simulink model "sgMdl_DNP3_1Client_1Server"  (R2024b)
settings: Solver=FixedStepAuto  StartTime=0.0  StopTime=inf  RelTol=1e-3  EnableMultiTasking=on
libraries: simulink x15, speedgoatlib_dnp3 x13
Description:
  | DNP3 - Loopback
settings Model: sg_rtwmakecfg_data=_sg_IO75X_v1_2_0__sg_netxLib_MSVC140_  ModifiedByFormat=Speedgoat  SimulationMode=external  Creator=Speedgoat  LastModifiedBy=Speedgoat
settings SolverCC: ConcurrentTasks=on  AlgebraicLoopSolver=TrustRegion  PositivePriorityOrder=on  InsertRTBMode=Never (minimum delay)
settings DataIOCC: LimitDataPoints=on  SaveFormat=StructureWithTime  ReturnWorkspaceOutputs=off
settings OptimizationCC: BlockReduction=off  BooleanDataType=off  OptimizeBlockIOStorage=off  BufferReuse=off  GlobalBufferReuse=off  ExpressionFolding=off  LocalBlockOutputs=off  OptimizeDataStoreBuffers=off  BusAssignmentInplaceUpdate=off
settings DebuggingCC: SaveWithParameterizedLinksMsg=none  UnderspecifiedInitializationDetection=Classic  MergeDetectMultiDrivingBlocksExec=none  SignalResolutionControl=TryResolveAllWithWarning  TasksWithSamePriorityMsg=none  ParameterOverflowMsg=warning  UnconnectedInputMsg=warning  UnconnectedOutputMsg=warning  UnconnectedLineMsg=warning  SFUnexpectedBacktrackingDiag=warning  SFNoUnconditionalDefaultTransitionDiag=warning  SFExecutionAtInitializationDiag=none  ArithmeticOperatorsInVariantConditions=warning
settings HardwareCC: ProdBitPerLong=64  ProdLongLongMode=on  ProdHWDeviceType=Intel->x86-64 (Linux 64)  TargetBitPerPointer=64  TargetBitPerSizeT=64  TargetBitPerPtrDiffT=64  TargetLongLongMode=on  TargetIntDivRoundTo=Zero  TargetEndianess=LittleEndian  TargetWordSize=64  TargetHWDeviceType=MATLAB Host
settings ModelReferenceCC: EnableRefExpFcnMdlSchedulingChecks=on  PropagateSignalLabelsOutOfModel=off
settings SFSimCC: SimUseLocalCustomCode=off  CustomCodeUndefinedFunction=UseInterfaceOnly
settings RTWCC: Description=Speedgoat Real-Time Target Machine  SystemTargetFile=speedgoat.tlc  TemplateMakefile=slrealtime_default_tmf  RTWUseLocalCustomCode=off  Toolchain=Simulink Real-Time Toolchain  BuildConfiguration=Faster Runs  TargetLang=C++  GPUComputeCapability=3.5  DLArmComputeVersion=19.05
settings CodeAppCC: StateflowObjectComments=on
settings SimulinkRealTimeTargetCC: SubcomponentCodeInterfacePackaging=Reusable function  InstructionSetFMA=off  LogToMDFFile=off  SLRTFileLogMaxRuns=10
settings ConfigComp: CovMetricSettings=dw  CovSaveCumulativeToWorkspaceVar=on  CovSaveSingleToWorkspaceVar=on  CovExternalEMLEnable=off  CovBoundaryAbsTol=1.0e-5

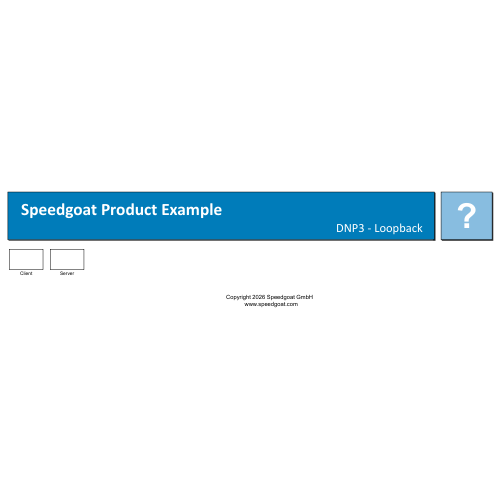
[thumbnail: Simulink's stored preview of the top-level diagram]
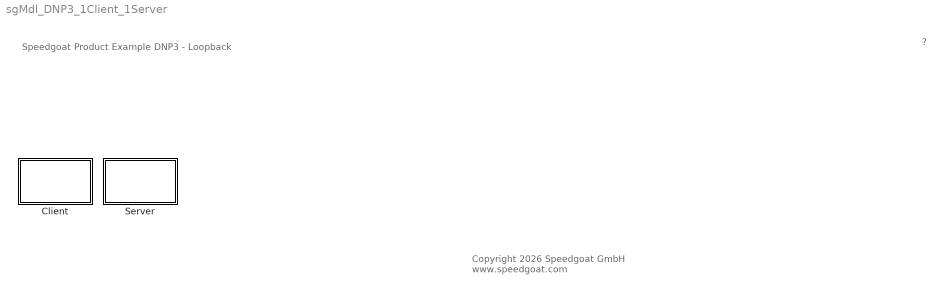
== system sgMdl_DNP3_1Client_1Server ==
  note: Speedgoat Product Example
      | DNP3 - Loopback
  note: ?
  note: Copyright 2026 Speedgoat GmbH
      |  www.speedgoat.com
  Client : Subsystem
  Server : Subsystem

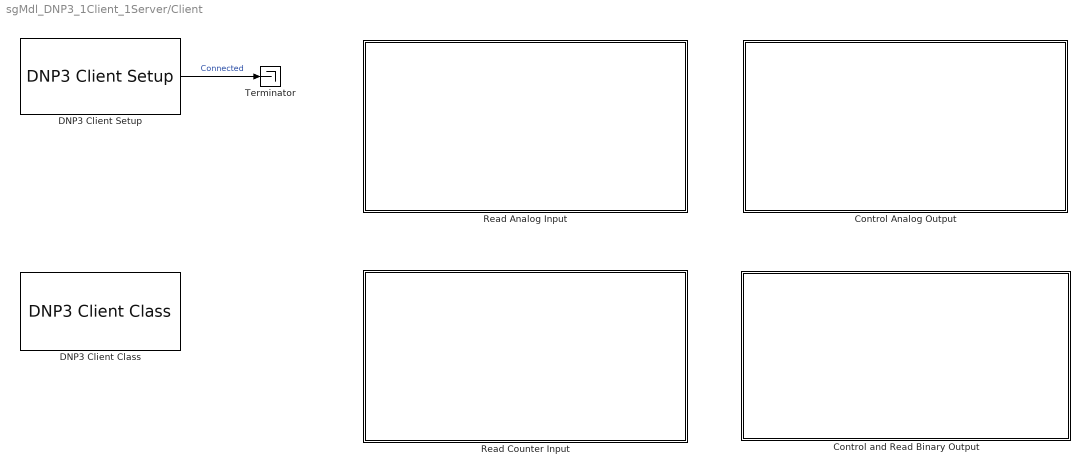
== system sgMdl_DNP3_1Client_1Server/Client ==
  Control Analog Output : Subsystem
  Control and Read Binary Output : Subsystem
  DNP3 Client Class : speedgoatlib_dnp3/Client/DNP3 Client Class  MasterID=0  OutstationID=1  SampleTime=-1  UnsolicitedClass0=off  UnsolicitedClass1=off  UnsolicitedClass2=off  UnsolicitedClass3=on  PollClass0=off  PollClass1=off  PollClass2=off  PollClass3=off  ClassTable={ '30 Analog input', '0', '1', 'Class 3' }
      settings: SourceProductName=DNP3
  DNP3 Client Setup : speedgoatlib_dnp3/Client/DNP3 Client Setup  NetworkID=0  MasterID=0  IpAddrStr='192.168.10.100'  KeepAlive=10000  RxTimeout=50  DataLinkRetries=3  SampleTime=0.001  OutstationTable={ '1', '192.168.10.101', '20000' }
      settings: SourceProductName=DNP3
  Read Analog Input : Subsystem
  Read Counter Input : Subsystem
  Terminator : Terminator
  wires:
  DNP3 Client Setup/1 -> Terminator/1  "Connected"

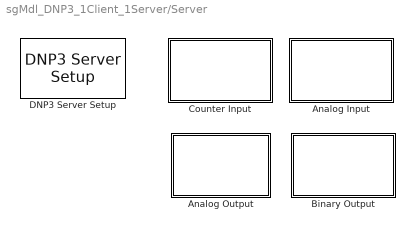
== system sgMdl_DNP3_1Client_1Server/Server ==
  Analog Input : Subsystem
  Analog Output : Subsystem
  Binary Output : Subsystem
  Counter Input : Subsystem
  DNP3 Server Setup : speedgoatlib_dnp3/Server/DNP3 Server Setup  OutstationID=1  IpAddrStr='192.168.10.101'  TcpPort=20000  Deadband=1.5  DevAttrCell={}  NumBinInPoints=8  NumBinInEvents=100  NumDBinInPoints=8  NumDBinInEvents=100  NumCntInPoints=8  NumCntInEvents=100  NumAnalogInPoints=8  NumAnalogInEvents=100  NumBinOutPoints=8  NumBinOutEvents=100  NumAnalogOutPoints=8  NumAnalogOutEvents=100
      settings: SourceProductName=DNP3

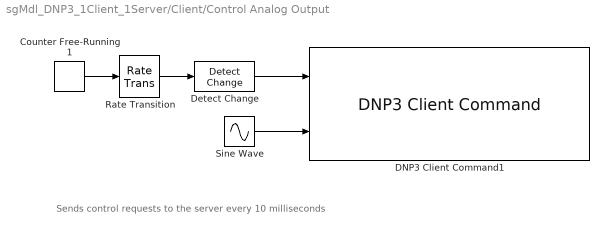
== system sgMdl_DNP3_1Client_1Server/Client/Control Analog Output ==
  note: Sends control requests to the server every 10 milliseconds
  Counter Free-Running1 : simulink/Sources/Counter Free-Running  NumBits=32  tsamp=0.01
  DNP3 Client Command1 : speedgoatlib_dnp3/Client/DNP3 Client Command  MasterID=0  OutstationID=1  CommandMode=Dropdown  CommandDropDown=41:04:05 Control analog output (64-bit float)  CommandEdit=[41 4 5]  Index=0  Quantity=1  SampleTime=0.001
      settings: AttributesFormatString=%<CommandDropdown>  SourceProductName=DNP3
  Detect Change : simulink/Logic and Bit Operations/Detect Change  vinit=0  OutDataTypeStr=boolean
  Rate Transition : RateTransition
  Sine Wave : Sin  SineType=Sample based  Amplitude=10  Samples=2000  SampleTime=0.001
  wires:
  Detect Change/1 -> DNP3 Client Command1/1
  Sine Wave/1 -> DNP3 Client Command1/2
  Counter Free-Running1/1 -> Rate Transition/1
  Rate Transition/1 -> Detect Change/1

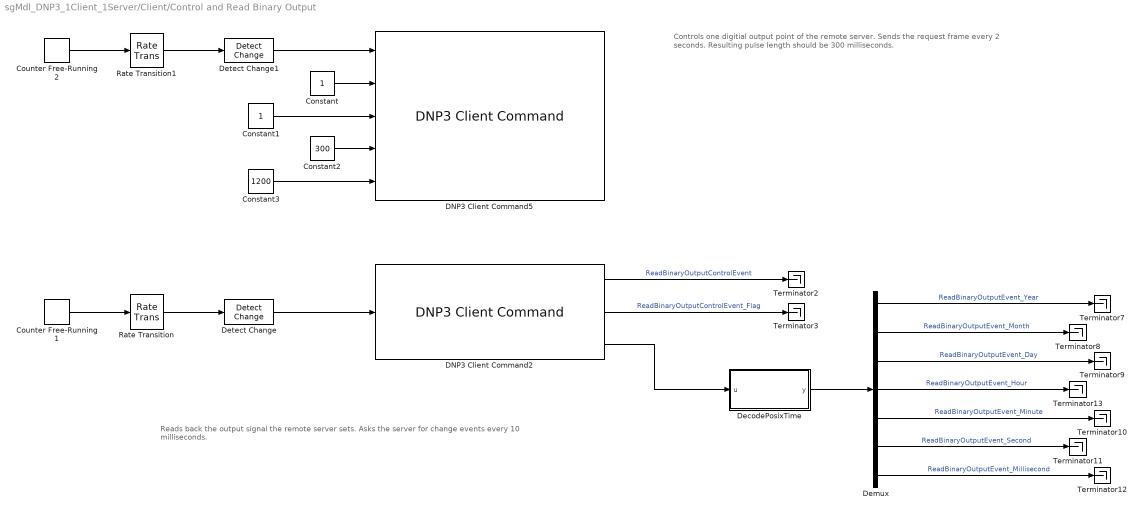
== system sgMdl_DNP3_1Client_1Server/Client/Control and Read Binary Output ==
  note: Controls one digitial output point of the remote server. Sends the request frame every 2 seconds. Resulting pulse length should be 300 milliseconds.
  note: Reads back the output signal the remote server sets. Asks the server for change events every 10 milliseconds.
  Constant : Constant  OutDataTypeStr=Inherit: Inherit via back propagation
  Constant1 : Constant  OutDataTypeStr=Inherit: Inherit via back propagation
  Constant2 : Constant  Value=300  OutDataTypeStr=Inherit: Inherit via back propagation
  Constant3 : Constant  Value=1200  OutDataTypeStr=Inherit: Inherit via back propagation
  Counter Free-Running1 : simulink/Sources/Counter Free-Running  NumBits=32  tsamp=0.01
  Counter Free-Running2 : simulink/Sources/Counter Free-Running  NumBits=32  tsamp=2
  DNP3 Client Command2 : speedgoatlib_dnp3/Client/DNP3 Client Command  MasterID=0  OutstationID=1  CommandMode=Dropdown  CommandDropDown=11:02:01 Read binary output event with time  CommandEdit=[11 2 1]  Index=0  Quantity=1  SampleTime=0.001
      settings: AttributesFormatString=%<CommandDropdown>  SourceProductName=DNP3
  DNP3 Client Command5 : speedgoatlib_dnp3/Client/DNP3 Client Command  MasterID=0  OutstationID=1  CommandMode=Dropdown  CommandDropDown=12:01:05 Control Relay Output  CommandEdit=[12 1 5]  Index=0  Quantity=1  SampleTime=0.001
      settings: AttributesFormatString=%<CommandDropdown>  SourceProductName=DNP3
  DecodePosixTime : MATLAB Function  TreatAsAtomicUnit=on
  Demux : Demux  Outputs=7
  Detect Change : simulink/Logic and Bit Operations/Detect Change  vinit=0  OutDataTypeStr=boolean
  Detect Change1 : simulink/Logic and Bit Operations/Detect Change  vinit=0  OutDataTypeStr=boolean
  Rate Transition : RateTransition
  Rate Transition1 : RateTransition
  Terminator{2..3,7..13} (9 alike) : Terminator
  wires:
  Demux/4 -> Terminator13/1  "ReadBinaryOutputEvent_Hour"
  Detect Change1/1 -> DNP3 Client Command5/1
  Constant1/1 -> DNP3 Client Command5/3
  Rate Transition1/1 -> Detect Change1/1
  Demux/3 -> Terminator9/1  "ReadBinaryOutputEvent_Day"
  Demux/5 -> Terminator10/1  "ReadBinaryOutputEvent_Minute"
  Counter Free-Running2/1 -> Rate Transition1/1
  Rate Transition/1 -> Detect Change/1
  Constant3/1 -> DNP3 Client Command5/5
  Demux/1 -> Terminator7/1  "ReadBinaryOutputEvent_Year"
  Constant2/1 -> DNP3 Client Command5/4
  Constant/1 -> DNP3 Client Command5/2
  Demux/2 -> Terminator8/1  "ReadBinaryOutputEvent_Month"
  Counter Free-Running1/1 -> Rate Transition/1
  DecodePosixTime/1(y) -> Demux/1
  DNP3 Client Command2/1 -> Terminator2/1  "ReadBinaryOutputControlEvent"
  DNP3 Client Command2/2 -> Terminator3/1  "ReadBinaryOutputControlEvent_Flag"
  Demux/7 -> Terminator12/1  "ReadBinaryOutputEvent_Millisecond"
  DNP3 Client Command2/3 -> DecodePosixTime/1(u)
  Demux/6 -> Terminator11/1  "ReadBinaryOutputEvent_Second"
  Detect Change/1 -> DNP3 Client Command2/1

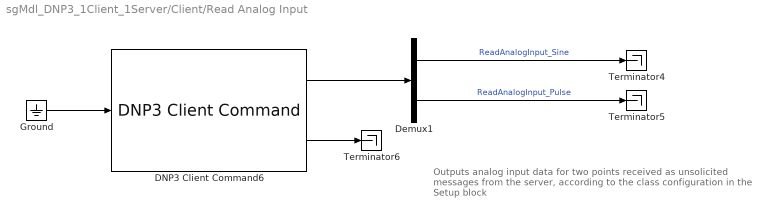
== system sgMdl_DNP3_1Client_1Server/Client/Read Analog Input ==
  note: Outputs analog input data for two points received as unsolicited messages from the server, according to the class configuration in the Setup block
  DNP3 Client Command6 : speedgoatlib_dnp3/Client/DNP3 Client Command  MasterID=0  OutstationID=1  CommandMode=Dropdown  CommandDropDown=32:06:01 Read analog input event with flag (64-bit float)  CommandEdit=[32 6 1]  Index=0  Quantity=2  SampleTime=0.001
      settings: AttributesFormatString=%<CommandDropdown>  SourceProductName=DNP3
  Demux1 : Demux  Outputs=2
  Ground : Ground
  Terminator4 : Terminator
  Terminator5 : Terminator
  Terminator6 : Terminator
  wires:
  Demux1/1 -> Terminator4/1  "ReadAnalogInput_Sine"
  Ground/1 -> DNP3 Client Command6/1
  Demux1/2 -> Terminator5/1  "ReadAnalogInput_Pulse"
  DNP3 Client Command6/2 -> Terminator6/1
  DNP3 Client Command6/1 -> Demux1/1

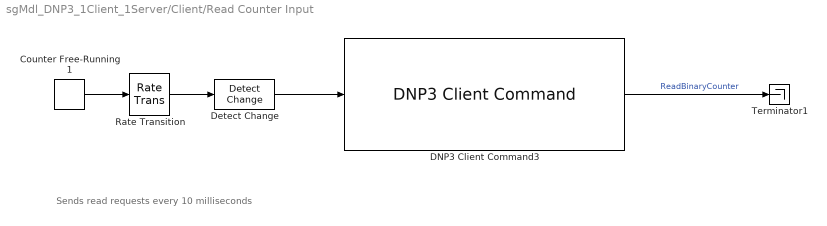
== system sgMdl_DNP3_1Client_1Server/Client/Read Counter Input ==
  note: Sends read requests every 10 milliseconds
  Counter Free-Running1 : simulink/Sources/Counter Free-Running  NumBits=32  tsamp=0.01
  DNP3 Client Command3 : speedgoatlib_dnp3/Client/DNP3 Client Command  MasterID=0  OutstationID=1  CommandMode=Dropdown  CommandDropDown=20:05:01 Read binary counter (32-bit integer)  CommandEdit=[20 5 1]  Index=0  Quantity=1  SampleTime=0.001
      settings: AttributesFormatString=%<CommandDropdown>  SourceProductName=DNP3
  Detect Change : simulink/Logic and Bit Operations/Detect Change  vinit=0  OutDataTypeStr=boolean
  Rate Transition : RateTransition
  Terminator1 : Terminator
  wires:
  DNP3 Client Command3/1 -> Terminator1/1  "ReadBinaryCounter"
  Detect Change/1 -> DNP3 Client Command3/1
  Counter Free-Running1/1 -> Rate Transition/1
  Rate Transition/1 -> Detect Change/1

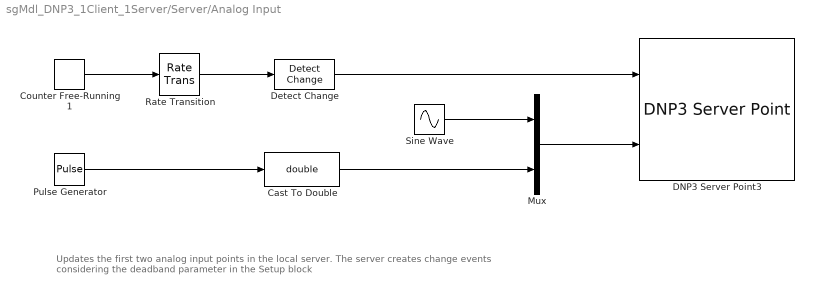
== system sgMdl_DNP3_1Client_1Server/Server/Analog Input ==
  note: Updates the first two analog input points in the local server. The server creates change events considering the deadband parameter in the Setup block
  Cast To Double : DataTypeConversion  OutDataTypeStr=double  SaturateOnIntegerOverflow=off  RndMeth=Floor
  Counter Free-Running1 : simulink/Sources/Counter Free-Running  NumBits=32  tsamp=0.01
  DNP3 Server Point3 : speedgoatlib_dnp3/Server/DNP3 Server Point  NetworkID=0  OutstationID=1  OperationMode=30 Write analog input  Length=2  SampleTime=0.001  Offset=0
      settings: AttributesFormatString=%<OperationMode>  SourceProductName=DNP3
  Detect Change : simulink/Logic and Bit Operations/Detect Change  vinit=0  OutDataTypeStr=boolean
  Mux : Mux  Inputs=2
  Pulse Generator : DiscretePulseGenerator  Amplitude=2  Period=1000  PulseWidth=500  SampleTime=0.001
  Rate Transition : RateTransition
  Sine Wave : Sin  SineType=Sample based  Amplitude=10  Samples=2000  SampleTime=0.001
  wires:
  Sine Wave/1 -> Mux/1
  Cast To Double/1 -> Mux/2
  Mux/1 -> DNP3 Server Point3/2
  Rate Transition/1 -> Detect Change/1
  Detect Change/1 -> DNP3 Server Point3/1
  Counter Free-Running1/1 -> Rate Transition/1
  Pulse Generator/1 -> Cast To Double/1

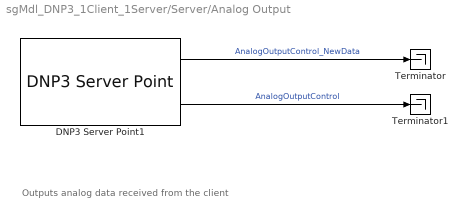
== system sgMdl_DNP3_1Client_1Server/Server/Analog Output ==
  note: Outputs analog data received from the client
  DNP3 Server Point1 : speedgoatlib_dnp3/Server/DNP3 Server Point  NetworkID=0  OutstationID=1  OperationMode=41 Indicate analog output control  Length=1  SampleTime=0.001  Offset=0
      settings: AttributesFormatString=%<OperationMode>  SourceProductName=DNP3
  Terminator : Terminator
  Terminator1 : Terminator
  wires:
  DNP3 Server Point1/2 -> Terminator1/1  "AnalogOutputControl"
  DNP3 Server Point1/1 -> Terminator/1  "AnalogOutputControl_NewData"

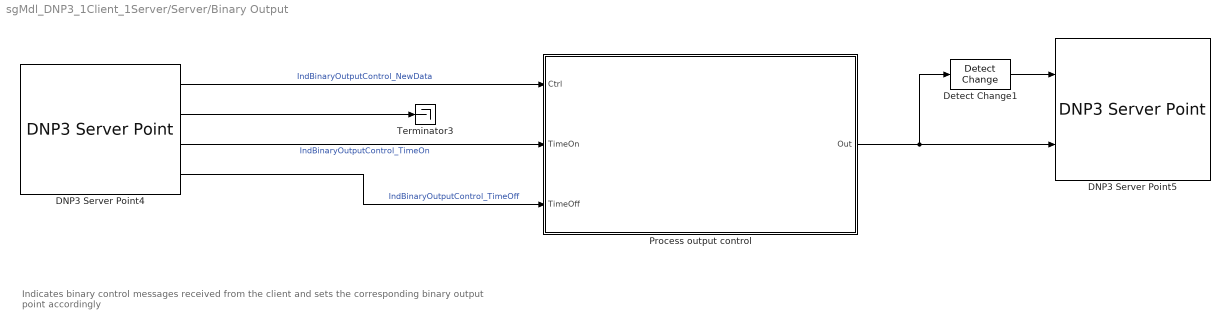
== system sgMdl_DNP3_1Client_1Server/Server/Binary Output ==
  note: Indicates binary control messages received from the client and sets the corresponding binary output point accordingly
  DNP3 Server Point4 : speedgoatlib_dnp3/Server/DNP3 Server Point  NetworkID=0  OutstationID=1  OperationMode=12 Indicate binary output control  Length=1  SampleTime=0.001  Offset=0
      settings: AttributesFormatString=%<OperationMode>  SourceProductName=DNP3
  DNP3 Server Point5 : speedgoatlib_dnp3/Server/DNP3 Server Point  NetworkID=0  OutstationID=1  OperationMode=10 Write binary output  Length=1  SampleTime=0.001  Offset=0
      settings: AttributesFormatString=%<OperationMode>  SourceProductName=DNP3
  Detect Change1 : simulink/Logic and Bit Operations/Detect Change  vinit=0  OutDataTypeStr=boolean
  Process output control : Subsystem
  Terminator3 : Terminator
  wires:
  DNP3 Server Point4/2 -> Terminator3/1
  DNP3 Server Point4/3 -> Process output control/2(TimeOn)  "IndBinaryOutputControl_TimeOn"
  DNP3 Server Point4/4 -> Process output control/3(TimeOff)  "IndBinaryOutputControl_TimeOff"
  Process output control/1(Out) -> Detect Change1/1, DNP3 Server Point5/2
  DNP3 Server Point4/1 -> Process output control/1(Ctrl)  "IndBinaryOutputControl_NewData"
  Detect Change1/1 -> DNP3 Server Point5/1

== system sgMdl_DNP3_1Client_1Server/Server/Counter Input ==
  note: Updates a local counter point
  Constant : Constant  OutDataTypeStr=Inherit: Inherit via back propagation
  Counter Free-Running : simulink/Sources/Counter Free-Running  NumBits=32  tsamp=0.001
  DNP3 Server Point2 : speedgoatlib_dnp3/Server/DNP3 Server Point  NetworkID=0  OutstationID=1  OperationMode=20 Write counter input  Length=1  SampleTime=0.001  Offset=0
      settings: AttributesFormatString=%<OperationMode>  SourceProductName=DNP3
  wires:
  Counter Free-Running/1 -> DNP3 Server Point2/2
  Constant/1 -> DNP3 Server Point2/1

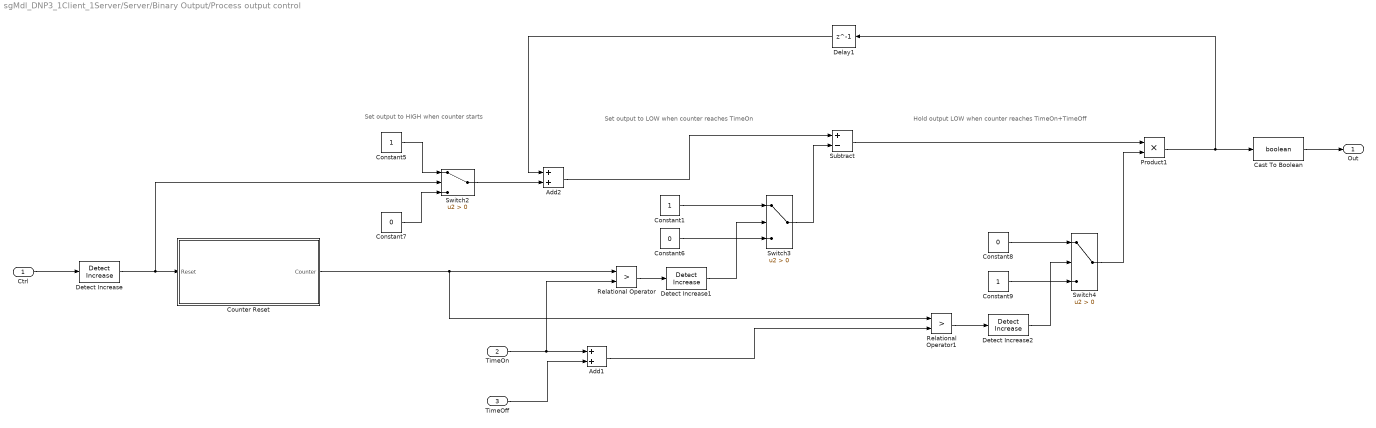
== system sgMdl_DNP3_1Client_1Server/Server/Binary Output/Process output control ==
  note: Hold output LOW when counter reaches TimeOn+TimeOff
  note: Set output to LOW when counter reaches TimeOn
  note: Set output to HIGH when counter starts
  Ctrl : Inport
  TimeOn : Inport  Port=2
  TimeOff : Inport  Port=3
  Add1 : Sum
  Add2 : Sum
  Cast To Boolean : DataTypeConversion  OutDataTypeStr=boolean  SaturateOnIntegerOverflow=off  RndMeth=Floor
  Constant1 : Constant
  Constant5 : Constant
  Constant6 : Constant  Value=0
  Constant7 : Constant  Value=0
  Constant8 : Constant  Value=0
  Constant9 : Constant
  Counter Reset : Subsystem
  Delay1 : Delay  DelayLength=1
  Detect Increase : simulink/Logic and Bit Operations/Detect Increase  vinit=0.0  OutDataTypeStr=boolean
  Detect Increase1 : simulink/Logic and Bit Operations/Detect Increase  vinit=0.0  OutDataTypeStr=boolean
  Detect Increase2 : simulink/Logic and Bit Operations/Detect Increase  vinit=0.0  OutDataTypeStr=boolean
  Product1 : Product
  Relational Operator : RelationalOperator  Operator=>  OutDataTypeStr=boolean  RndMeth=Simplest  InputSameDT=off
  Relational Operator1 : RelationalOperator  Operator=>  OutDataTypeStr=boolean  RndMeth=Simplest  InputSameDT=off
  Subtract : Sum  Inputs=+-
  Switch2 : Switch  Criteria=u2 > Threshold  SaturateOnIntegerOverflow=off  InputSameDT=off
  Switch3 : Switch  Criteria=u2 > Threshold  SaturateOnIntegerOverflow=off  InputSameDT=off
  Switch4 : Switch  Criteria=u2 > Threshold  SaturateOnIntegerOverflow=off  InputSameDT=off
  Out : Outport
  wires:
  Constant6/1 -> Switch3/3
  Detect Increase/1 -> Switch2/2, Counter Reset/1(Reset)
  Delay1/1 -> Add2/1
  Constant9/1 -> Switch4/3
  Constant1/1 -> Switch3/1
  Detect Increase2/1 -> Switch4/2
  Product1/1 -> Cast To Boolean/1, Delay1/1
  Add1/1 -> Relational Operator1/2
  Switch3/1 -> Subtract/2
  Subtract/1 -> Product1/1
  Add2/1 -> Subtract/1
  Relational Operator/1 -> Detect Increase1/1
  Relational Operator1/1 -> Detect Increase2/1
  Switch4/1 -> Product1/2
  Switch2/1 -> Add2/2
  Detect Increase1/1 -> Switch3/2
  Constant8/1 -> Switch4/1
  TimeOn/1 -> Relational Operator/2, Add1/1
  Ctrl/1 -> Detect Increase/1
  Constant5/1 -> Switch2/1
  Constant7/1 -> Switch2/3
  TimeOff/1 -> Add1/2
  Counter Reset/1(Counter) -> Relational Operator1/1, Relational Operator/1
  Cast To Boolean/1 -> Out/1

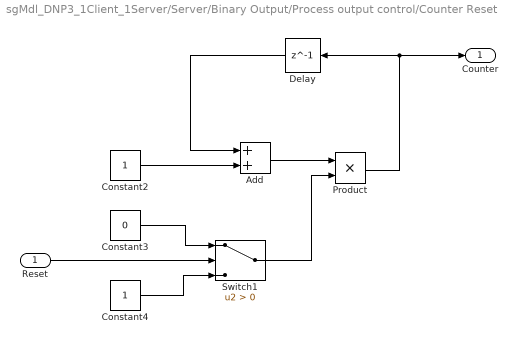
== system sgMdl_DNP3_1Client_1Server/Server/Binary Output/Process output control/Counter Reset ==
  Reset : Inport
  Add : Sum
  Constant2 : Constant
  Constant3 : Constant  Value=0
  Constant4 : Constant
  Delay : Delay  DelayLength=1
  Product : Product
  Switch1 : Switch  Criteria=u2 > Threshold  SaturateOnIntegerOverflow=off  InputSameDT=off
  Counter : Outport
  wires:
  Add/1 -> Product/1
  Constant4/1 -> Switch1/3
  Delay/1 -> Add/1
  Reset/1 -> Switch1/2
  Product/1 -> Counter/1, Delay/1
  Constant2/1 -> Add/2
  Switch1/1 -> Product/2
  Constant3/1 -> Switch1/1

== matlab function sgMdl_DNP3_1Client_1Server/Client/Control and Read Binary Output/DecodePosixTime ==
  data: u input; y output
function y = fcn(u)

y = zeros(1,7);
y(1,1:6) = datevec(datetime(floor(u/1000),'ConvertFrom','posixtime'));
y(7) = mod(u,uint64(1000));
